simulink model "AdaptivePacing"  (R2020a)
settings: Solver=FixedStepAuto  StartTime=0.0  StopTime=inf  FixedStep=1e-3  RelTol=1e-3  EnableMultiTasking=on
libraries: frdmk64flib x2
settings Model: ExtModeTrigDuration=5  Creator=amrad  LastModifiedBy=iceca
settings OptimizationCC: EnhancedBackFolding=on  PassReuseOutputArgsAs=Individual arguments  ZeroExternalMemoryAtStartup=off  ZeroInternalMemoryAtStartup=off  MaxStackSize=64  OptimizeBlockOrder=speed  DifferentSizesBufferReuse=on  OptimizationCustomize=off  EfficientTunableParamExpr=on
settings DebuggingCC: ParameterTunabilityLossMsg=error
settings HardwareCC: ProdBitPerPointer=32  ProdBitPerSizeT=32  ProdBitPerPtrDiffT=32  ProdLargestAtomicInteger=Long  ProdLargestAtomicFloat=Double  ProdWordSize=32  ProdHWDeviceType=ARM Compatible->ARM Cortex
settings SFSimCC: MATLABDynamicMemAlloc=off
settings RTWCC: SystemTargetFile=ert.tlc  HardwareBoard=NXP FRDM-K64F  TemplateMakefile=ert_default_tmf  Toolchain=GNU Tools for ARM Embedded Processors
settings CodeAppCC: ForceParamTrailComments=on  IgnoreCustomStorageClasses=off  OperatorAnnotations=on  SimulinkDataObjDesc=on  SFDataObjDesc=on  InsertBlockDesc=on

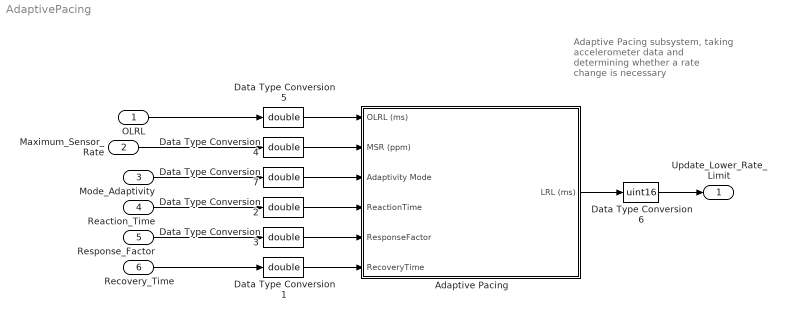
== system AdaptivePacing ==
  note: Adaptive Pacing subsystem, taking accelerometer data and determining whether a rate change is necessary
  OLRL : Inport  OutDataTypeStr=uint16
  Maximum_Sensor_Rate : Inport  Port=2  OutDataTypeStr=uint8
  Mode_Adaptivity : Inport  Port=3  OutDataTypeStr=uint8
  Reaction_Time : Inport  Port=4  OutDataTypeStr=uint8
  Response_Factor : Inport  Port=5  OutDataTypeStr=uint8
  Recovery_Time : Inport  Port=6  OutDataTypeStr=uint8
  Adaptive Pacing : Subsystem
  Data Type Conversion{1..5,7} (6 alike) : DataTypeConversion  OutDataTypeStr=double
  Data Type Conversion6 : DataTypeConversion  OutDataTypeStr=uint16
  Update_Lower_Rate_Limit : Outport
  wires:
  Data Type Conversion3/1 -> Adaptive Pacing/5(ResponseFactor)
  Data Type Conversion7/1 -> Adaptive Pacing/3(Adaptivity Mode)
  Data Type Conversion2/1 -> Adaptive Pacing/4(ReactionTime)
  Data Type Conversion1/1 -> Adaptive Pacing/6(RecoveryTime)
  OLRL/1 -> Data Type Conversion5/1
  Reaction_Time/1 -> Data Type Conversion2/1
  Data Type Conversion5/1 -> Adaptive Pacing/1(OLRL (ms))
  Maximum_Sensor_Rate/1 -> Data Type Conversion4/1
  Mode_Adaptivity/1 -> Data Type Conversion7/1
  Recovery_Time/1 -> Data Type Conversion1/1
  Data Type Conversion4/1 -> Adaptive Pacing/2(MSR (ppm))
  Adaptive Pacing/1(LRL (ms)) -> Data Type Conversion6/1
  Response_Factor/1 -> Data Type Conversion3/1
  Data Type Conversion6/1 -> Update_Lower_Rate_Limit/1

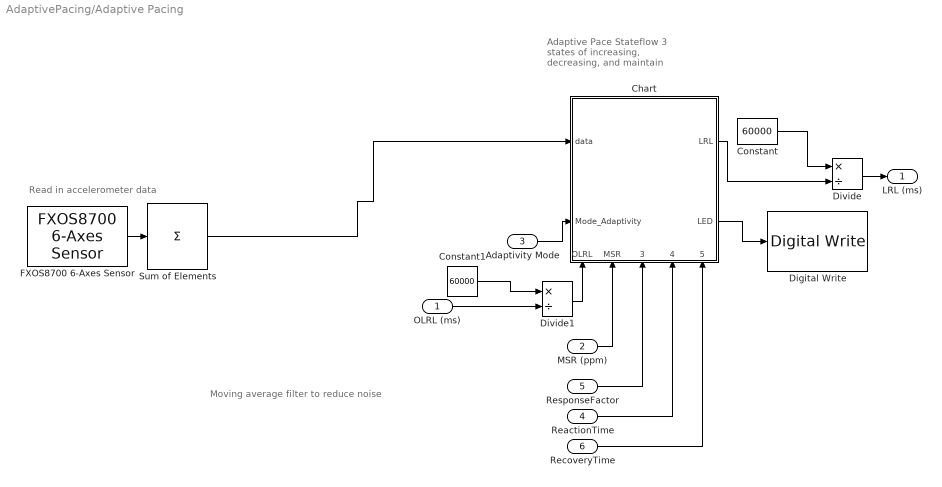
== system AdaptivePacing/Adaptive Pacing ==
  note: Moving average filter to reduce noise
  note: Read in accelerometer data
  note: Adaptive Pace Stateflow 3 states of increasing, decreasing, and maintain
  OLRL (ms) : Inport
  MSR (ppm) : Inport  Port=2
  Adaptivity Mode : Inport  Port=3
  ReactionTime : Inport  Port=4
  ResponseFactor : Inport  Port=5
  RecoveryTime : Inport  Port=6
  Chart : Stateflow chart  TreatAsAtomicUnit=on
      settings: PortSchema="{\"entries\":[{\"content\":{\"sides\":[{\"content\":{\"connectorIds\":[\"In6\",\"In7\"]},\"type\":\"ConnectorPlacement.EquallySpacedRectSide\",\"uuid\":\"5e590210-4b26-43ca-b410-899265592776\"},{\"content\":{\"connectorIds\":[\"Out1\",\"Out2\"],\"side\":\"RIGHT\"},\"type\":\"ConnectorPlacement.EquallySpacedRectSide\",\"uuid\":\"99d9f5d1-b5a6-4f8b-b4f2-efe260ebc8c4\"},{\"content\":{\"connectorIds\":[],\"side\":\"TOP\"},\"type\":\"ConnectorPlacement.EquallySpacedRectSide\",\"uuid\":\"3c56162d-1f91-43ab-bf8d-9a1cf5be554c\"},{\"content\":{\"connectorIds\":[\"In1\",\"In2\",\"In3\",\"In4\",\"In5\"],\"side\":\"BOTTOM\"},\"type\":\"ConnectorPlacement.EquallySpacedRectSide\",\"uuid\":\"2e827a33-e1bf-40db-bbb6-314ece1f4eba\"}]},\"type\":\"ConnectorPlacement.EquallySpacedConnector\",\"uuid\":\"7a7dbe64-1607-48a8-bc2e-dcaf5b987588\"}],\"packageUris\":[\"http://schema.mathworks.com/mf0/Connector/19700101\"],\"version\":\"1.0\"}"
  Constant : Constant  Value=60000  SampleTime=-1
  Constant1 : Constant  Value=60000  SampleTime=-1
  Digital Write : frdmk64flib/Digital Write  Whichpin=RED_LED
  Divide : Product  Inputs=*/
  Divide1 : Product  Inputs=*/
  FXOS8700 6-Axes Sensor : frdmk64flib/FXOS8700 6-Axes Sensor  Activesensor=Accelerometer only  ODR=800Hz  HybridODR=400Hz  Accelfullrange=-2g to +2g  SampleTime=-1
  Sum of Elements : Sum  Inputs=+
  LRL (ms) : Outport
  wires:
  FXOS8700 6-Axes Sensor/1 -> Sum of Elements/1
  ResponseFactor/1 -> Chart/3(ResponseFactor)
  MSR (ppm)/1 -> Chart/2(MSR)
  ReactionTime/1 -> Chart/4(reactionTime)
  RecoveryTime/1 -> Chart/5(recoveryTime)
  Chart/1(LRL) -> Divide/2
  Divide/1 -> LRL (ms)/1
  OLRL (ms)/1 -> Divide1/2
  Divide1/1 -> Chart/1(OLRL)
  Constant/1 -> Divide/1
  Adaptivity Mode/1 -> Chart/7(Mode_Adaptivity)
  Sum of Elements/1 -> Chart/6(data)
  Constant1/1 -> Divide1/1
  Chart/2(LED) -> Digital Write/1

== stateflow chart AdaptivePacing/Adaptive Pacing/Chart ==
  state start
    entry:
    LRL=OLRL;
    RateChange=ResponseFactor/16;
    Avg = 0;
  note: Increase the LRL is mode adaptivity
  note: Only increase the rate if mode adaptivity.
  state main
    entry:
    %not a moving average window, but a exponential window
    Avg = Avg*0.7+data*0.3;
    %make sure LRL never exceeds MSR or goes below MSR
    LRL = max(OLRL, LRL);
    LRL=min(LRL, MSR);
  state Increasing
    entry:
    LRL=LRL+RateChange;
  state Constant
    entry:
    LRL=OLRL;
    LED=true;
  state Decreasing
    entry:
    LRL=LRL-RateChange;
  (default) -> start
  start -> main
  main -> Increasing [order 2] : [Mode_Adaptivity==1 && data>1.05 && LRL<MSR]
  Constant -> main
  Increasing -> main : [after(reactionTime,msec)]
  main -> Constant [order 3] : [Mode_Adaptivity==0]
  Decreasing -> main : [after(recoveryTime,msec)]
  main -> Decreasing [order 1] : [Mode_Adaptivity==1 && data<1.05 && LRL>OLRL]
  data: OLRL input; MSR input; ResponseFactor input; reactionTime input; recoveryTime input; data input; LRL output double; RateChange local; Avg local; Mode_Adaptivity input; LED output
